simulink model "model_simulink"  (R2023b)
settings: Solver=VariableStepAuto  StartTime=0.0  StopTime=t_final  RelTol=1e-3
values from neighbouring files (symbols this model uses):
  A = 0.4884    [Percetual_influence.m]    (also in model.m = 0.28432)
  bikeChoice = menu('Choose a Bike', 'Phoenix', 'Taurus', 'Cerberus')    [Percetual_influence.m]    (also in model.m)
  crr_1 = 0.0012    [Percetual_influence.m]    (also in model.m)
  crr_2 = 0.000038    (= 3.8e-05)    [Percetual_influence.m]    (also in model.m)
  Cx_vec = [0.0438 0.0404 0.0385 0.0364 0.0349 0.0337 0.0329 0.0326 0.0325 0.0324 0.0326]    [Percetual_influence.m]    (also in model.m = [0.04047 0.03601 0.03308 0.03102 0.02973 0.03069 0.03548 0.0)
  CxA_ref = 0.01836    [Percetual_influence.m]    (also in model.m)
  eta_tot = 0.97    [Percetual_influence.m]    (also in model.m)
  g = 9.81    [Percetual_influence.m]    (also in model.m)
  L = 2.80    (= 2.8)    [Percetual_influence.m]    (also in model.m)
  m = mv+mr+mw    (= 102.5)    [Percetual_influence.m]    (also in model.m)
  me = mr+mv+mw*1.5    (= 104.75)    [Percetual_influence.m]    (also in model.m)
  mu = 0.0000198    (= 1.98e-05)    [Percetual_influence.m]    (also in model.m)
  n_start = 0    [Percetual_influence.m]    (also in model.m)
  R_wheel = 0.235    [Percetual_influence.m]    (also in model.m = 0.23157)
  rho = 0.97    [Percetual_influence.m]    (also in model.m)
  v_init = Speed_vector(2)/3.6    [Percetual_influence.m]    (also in model.m)
  v_ref = 27.78    [Percetual_influence.m]    (also in model.m)
  V_vec = [30:10:100 105:5:115]/3.6    [Percetual_influence.m]    (also in model.m = [30:10:100 105:5:150]/3.6)
libraries: simulink_extras x1
settings Model: Creator=mac  LastModifiedBy=matti
settings DataIOCC: SignalLogging=off  DSMLogging=off  SaveTime=off  ReturnWorkspaceOutputs=off

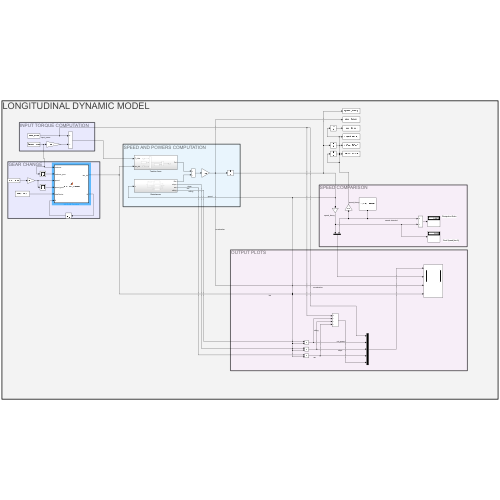
[thumbnail: Simulink's stored preview of the top-level diagram]
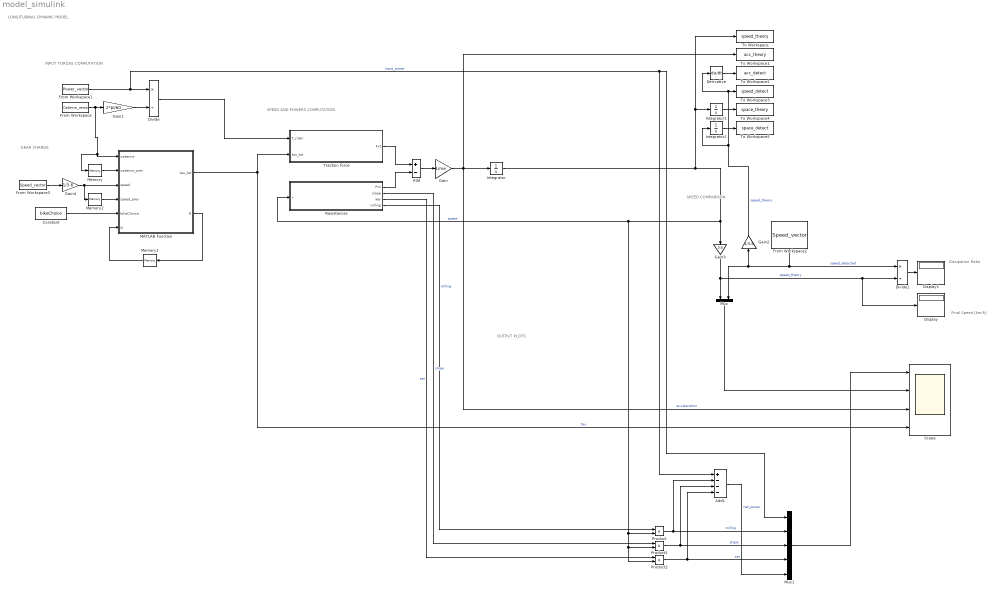
== system model_simulink ==
  note: LONGITUDINAL DYNAMIC MODEL
  note: OUTPUT PLOTS
  note: SPEED COMPARISON
  note: SPEED AND POWERS COMPUTATION
  note: INPUT TORQUE COMPUTATION
  note: GEAR CHANGE
  note: Final Speed [km/h]
  note: Dissipation Ratio
  Add : Sum  Inputs=+-
  Add1 : Sum  Inputs=+---
  Constant : Constant  Value=bikeChoice
  Derivative : Derivative
  Display : Display
  Display1 : Display
  Divide : Product  Inputs=*/
  Divide1 : Product  Inputs=*/
  From Workspace : FromWorkspace  VariableName=Cadence_vector  OutDataTypeStr=double  SampleTime=-1
  From Workspace1 : FromWorkspace  VariableName=Power_vector  OutDataTypeStr=double  SampleTime=-1
  From Workspace2 : FromWorkspace  VariableName=Speed_vector
  From Workspace3 : FromWorkspace  VariableName=Speed_vector  OutDataTypeStr=double  SampleTime=-1
  Gain : Gain  Gain=1/me
  Gain1 : Gain  Gain=2*pi/60
  Gain2 : Gain  Gain=1/3.6
  Gain3 : Gain  Gain=3.6
  Gain4 : Gain  Gain=1/3.6
  Integrator : Integrator  InitialCondition=v_init
  Integrator1 : Integrator
  Integrator2 : Integrator
  MATLAB Function : MATLAB Function  TreatAsAtomicUnit=on
  Memory : Memory
  Memory1 : Memory  InitialCondition=n_start
  Memory2 : Memory
  Mux : Mux  Inputs=2
  Mux1 : Mux  Inputs=5
  Product : Product
  Product1 : Product
  Product2 : Product
  Resistances : Subsystem
  Scope : Scope  NumInputPorts=4
  To Workspace : ToWorkspace  VariableName=speed_theory  SaveFormat=Timeseries  SampleTime=-1
      settings: Save2DSignal=2-D array (concatenate along first dimension)
  To Workspace1 : ToWorkspace  VariableName=acc_theory  SaveFormat=Timeseries  SampleTime=-1
      settings: Save2DSignal=2-D array (concatenate along first dimension)
  To Workspace2 : ToWorkspace  VariableName=acc_detect  SaveFormat=Timeseries  SampleTime=-1
      settings: Save2DSignal=2-D array (concatenate along first dimension)
  To Workspace3 : ToWorkspace  VariableName=speed_detect  SaveFormat=Timeseries  SampleTime=-1
      settings: Save2DSignal=2-D array (concatenate along first dimension)
  To Workspace4 : ToWorkspace  VariableName=space_theory  SaveFormat=Timeseries  SampleTime=-1
      settings: Save2DSignal=2-D array (concatenate along first dimension)
  To Workspace5 : ToWorkspace  VariableName=space_detect  SaveFormat=Timeseries  SampleTime=-1
      settings: Save2DSignal=2-D array (concatenate along first dimension)
  Traction force : Subsystem
  wires:
  Traction force/1(Fxt) -> Add/1
  Resistances/1(Rm) -> Add/2
  Add/1 -> Gain/1
  Gain/1 -> To Workspace1/1, Scope/3, Integrator/1  "acceleration"
  Integrator/1 -> Integrator1/1, To Workspace/1, Gain3/1, Resistances/1(v), Product/2, Product1/2, Product2/2  "speed"
  Divide/1 -> Traction force/1(T_rider)
  Gain1/1 -> Divide/2
  From Workspace/1 -> MATLAB Function/1(cadence), Memory/1, Gain1/1
  MATLAB Function/1(tau_tot) -> Traction force/2(tau_tot), Scope/4  "tau"
  Memory/1 -> MATLAB Function/2(cadence_prev)
  MATLAB Function/2(N) -> Memory1/1
  Memory1/1 -> MATLAB Function/6("N ")
  Resistances/2(slope) -> Product1/1  "slope"
  Resistances/3(aer) -> Product2/1  "aer"
  Resistances/4(rolling) -> Product/1  "rolling"
  Product/1 -> Add1/2, Mux1/2  "rolling"
  Mux1/1 -> Scope/1
  Product1/1 -> Mux1/3, Add1/3  "slope"
  Product2/1 -> Mux1/4, Add1/4  "aer"
  Add1/1 -> Mux1/5  "net_power"
  Gain3/1 -> Divide1/2, Display/1, Mux/1  "speed_theory"
  From Workspace2/1 -> Gain2/1, Mux/2, Divide1/1  "speed_detected"
  Mux/1 -> Scope/2
  Divide1/1 -> Display1/1
  From Workspace1/1 -> Divide/1, Add1/1, Mux1/1  "input_power"
  Gain2/1 -> Integrator2/1, Derivative/1, To Workspace3/1  "speed_theory"
  Derivative/1 -> To Workspace2/1
  Integrator1/1 -> To Workspace4/1
  Integrator2/1 -> To Workspace5/1
  From Workspace3/1 -> Gain4/1
  Memory2/1 -> MATLAB Function/4(speed_prev)
  Gain4/1 -> Memory2/1, MATLAB Function/3(speed)
  Constant/1 -> MATLAB Function/5(bikeChoice)

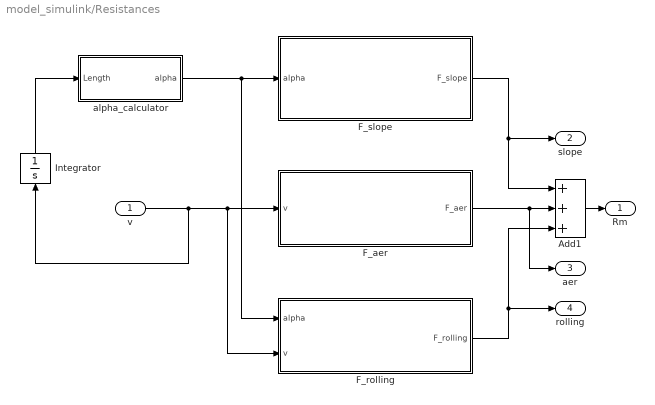
== system model_simulink/Resistances ==
  v : Inport
  Add1 : Sum  Inputs=+++
  F_aer : Subsystem
  F_rolling : Subsystem
  F_slope : Subsystem
  Integrator : Integrator
  alpha_calculator : Subsystem
  Rm : Outport
  slope : Outport  Port=2
  aer : Outport  Port=3
  rolling : Outport  Port=4
  wires:
  F_slope/1(F_slope) -> slope/1, Add1/1
  v/1 -> Integrator/1, F_aer/1(v), F_rolling/2(v)
  Add1/1 -> Rm/1
  F_rolling/1(F_rolling) -> rolling/1, Add1/3
  F_aer/1(F_aer) -> aer/1, Add1/2
  alpha_calculator/1(alpha) -> F_rolling/1(alpha), F_slope/1(alpha)
  Integrator/1 -> alpha_calculator/1(Length)

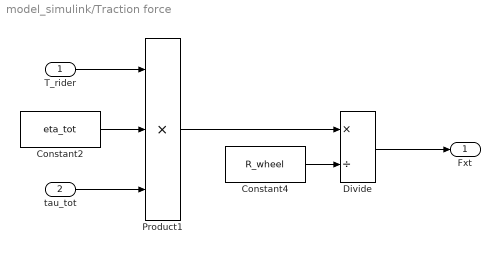
== system model_simulink/Traction force ==
  T_rider : Inport
  tau_tot : Inport  Port=2
  Constant2 : Constant  Value=eta_tot
  Constant4 : Constant  Value=R_wheel
  Divide : Product  Inputs=*/
  Product1 : Product  Inputs=3
  Fxt : Outport
  wires:
  T_rider/1 -> Product1/1
  Constant4/1 -> Divide/2
  Product1/1 -> Divide/1
  Divide/1 -> Fxt/1
  tau_tot/1 -> Product1/3
  Constant2/1 -> Product1/2

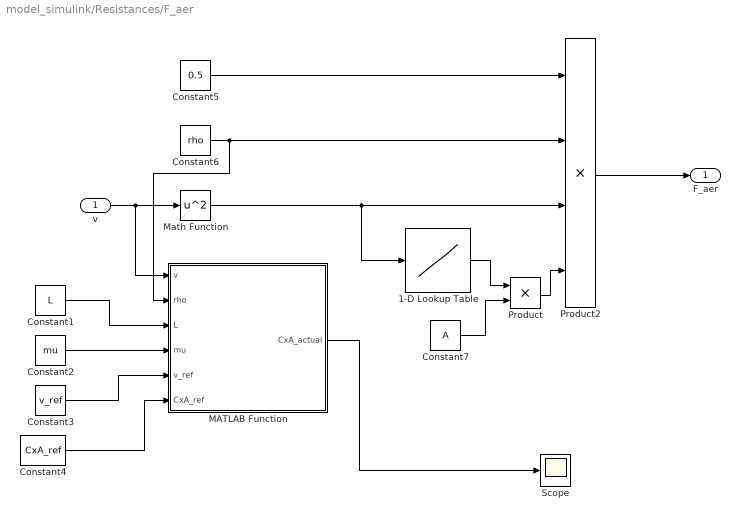
== system model_simulink/Resistances/F_aer ==
  v : Inport
  1-D Lookup Table : Lookup_n-D  NumberOfTableDimensions=1  BreakpointsForDimension1=V_vec  Table=Cx_vec  InternalRulePriority=Speed  RndMeth=Simplest
  Constant1 : Constant  Value=L
  Constant2 : Constant  Value=mu
  Constant3 : Constant  Value=v_ref
  Constant4 : Constant  Value=CxA_ref
  Constant5 : Constant  Value=0.5
  Constant6 : Constant  Value=rho
  Constant7 : Constant  Value=A
  MATLAB Function : MATLAB Function  TreatAsAtomicUnit=on
  Math Function : Math  Operator=square
  Product : Product
  Product2 : Product  Inputs=4
  Scope : Scope
  F_aer : Outport
  wires:
  Constant6/1 -> MATLAB Function/2(rho), Product2/2
  Constant5/1 -> Product2/1
  MATLAB Function/1(CxA_actual) -> Scope/1
  Product2/1 -> F_aer/1
  v/1 -> MATLAB Function/1(v), Math Function/1
  Constant1/1 -> MATLAB Function/3(L)
  Constant2/1 -> MATLAB Function/4(mu)
  Constant3/1 -> MATLAB Function/5(v_ref)
  Constant4/1 -> MATLAB Function/6(CxA_ref)
  Constant7/1 -> Product/2
  1-D Lookup Table/1 -> Product/1
  Math Function/1 -> 1-D Lookup Table/1, Product2/3
  Product/1 -> Product2/4

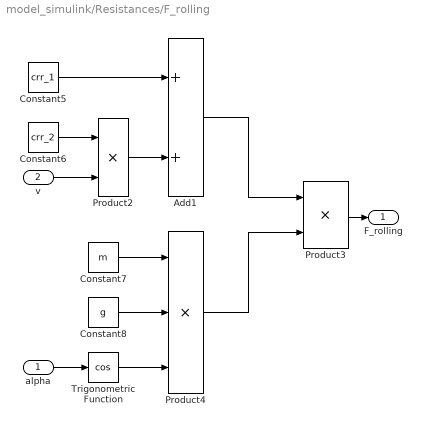
== system model_simulink/Resistances/F_rolling ==
  alpha : Inport
  v : Inport  Port=2
  Add1 : Sum
  Constant5 : Constant  Value=crr_1
  Constant6 : Constant  Value=crr_2
  Constant7 : Constant  Value=m
  Constant8 : Constant  Value=g
  Product2 : Product
  Product3 : Product
  Product4 : Product  Inputs=3
  Trigonometric Function : Trigonometry  Operator=cos
  F_rolling : Outport
  wires:
  Constant5/1 -> Add1/1
  Product3/1 -> F_rolling/1
  Constant6/1 -> Product2/1
  v/1 -> Product2/2
  Product2/1 -> Add1/2
  Trigonometric Function/1 -> Product4/3
  Constant7/1 -> Product4/1
  Constant8/1 -> Product4/2
  Product4/1 -> Product3/2
  alpha/1 -> Trigonometric Function/1
  Add1/1 -> Product3/1

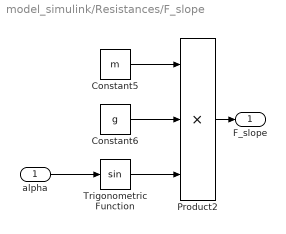
== system model_simulink/Resistances/F_slope ==
  alpha : Inport
  Constant5 : Constant  Value=m
  Constant6 : Constant  Value=g
  Product2 : Product  Inputs=3
  Trigonometric Function : Trigonometry
  F_slope : Outport
  wires:
  Constant6/1 -> Product2/2
  Product2/1 -> F_slope/1
  Constant5/1 -> Product2/1
  Trigonometric Function/1 -> Product2/3
  alpha/1 -> Trigonometric Function/1

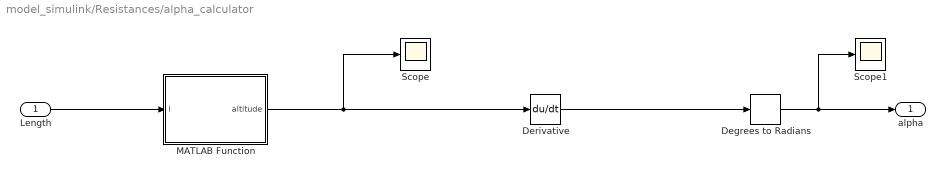
== system model_simulink/Resistances/alpha_calculator ==
  Length : Inport
  Degrees to Radians : simulink_extras/Transformations/Degrees to Radians
  Derivative : Derivative
  MATLAB Function : MATLAB Function  TreatAsAtomicUnit=on
  Scope : Scope
  Scope1 : Scope
  alpha : Outport
  wires:
  Degrees to Radians/1 -> alpha/1, Scope1/1
  Length/1 -> MATLAB Function/1(l)
  MATLAB Function/1(altitude) -> Scope/1, Derivative/1
  Derivative/1 -> Degrees to Radians/1

== matlab function model_simulink/MATLAB Function ==
  data: cadence input; tau_tot output; cadence_prev input; speed input; speed_prev input; bikeChoice input; N output; N input
function [tau_tot,N]  = GearChangeDetect(cadence,cadence_prev,speed,speed_prev, bikeChoice, N)
T = 1;

if bikeChoice == 1

% Verifica quando i valori cominciano a diminuire
if  cadence <= cadence_prev &&  speed >= speed_prev
    % Imposta un cambio marcia in su
    N = N+1;
else
    N = N;  % Mantieni la stessa marcia
end

n = N;

    if n == 12
        T = 12;
    elseif n == 11
        T = 13;
    elseif n == 10
        T = 14;
    elseif n == 9
        T = 15;
    elseif n == 8
        T = 17;
    elseif n == 7
        T = 19;
    elseif n == 6
        T = 21;
    elseif n == 5
        T = 24;
    elseif n == 4
        T = 27;
    elseif n == 3
        T = 31;
    elseif n == 2
        T = 35;
    elseif n == 1
        T = 40;
    elseif n > 12
        T = 12;
    else
        T = 40;
    end

tau_tot = (T/108)*(18/38);


elseif bikeChoice == 2
    % Verifica quando i valori cominciano a diminuire
if  cadence <= cadence_prev &&  speed >= speed_prev
    % Imposta un cambio marcia in su
    N = N+1;
else
    N = N;  % Mantieni la stessa marcia
end

n = N;

    if n == 12
        T = 12;
    elseif n == 11
        T = 13;
    elseif n == 10
        T = 14;
    elseif n == 9
        T = 15;
    elseif n == 8
        T = 17;
    elseif n == 7
        T = 19;
    elseif n == 6
        T = 21;
    elseif n == 5
        T = 24;
    elseif n == 4
        T = 27;
    elseif n == 3
        T = 31;
    elseif n == 2
        T = 35;
    elseif n == 1
        T = 40;
    elseif n > 12
        T = 12;
    else
        T = 40;
    end

tau_tot = (T/108)*(18/38);

else
    % Verifica quando i valori cominciano a diminuire
if  cadence <= 0.999 * cadence_prev &&  speed >= speed_prev
    % Imposta un cambio marcia in su
    N = N+1;
else
    N = N;  % Mantieni la stessa marcia
end

nc = N;

    if nc == 7
        T = 15;
    elseif nc == 6
        T = 17;
    elseif nc == 5
        T = 19;
    elseif nc == 4
        T = 21;
    elseif nc == 3
        T = 24;
    elseif nc == 2
        T = 28;
    elseif nc == 1
        T = 32;
    elseif nc > 7
        T = 15;
    else
        T = 32;
    end

tau_tot = (T/60)*(17/54);

end

== matlab function model_simulink/Resistances/F_aer/MATLAB Function ==
  data: v input; CxA_actual output; rho input; L input; mu input; v_ref input; CxA_ref input
function CxA_actual = fcn(v,rho,L,mu,v_ref,CxA_ref)

Re = v*rho*L/mu;
Vect = [0.074*(Re^-0.2),0.01];
Num = min(Vect);
Den = 0.074*((v_ref*rho*L/mu)^-0.2);

CxA_actual = CxA_ref*Num/Den;

== matlab function model_simulink/Resistances/alpha_calculator/MATLAB Function ==
  data: l input; altitude output
function altitude = fcn(l)

altitude = -5.93e-15*l^4+2.22e-10*l^3-2.349e-06*l^2+0.003799*l+31.33;

end
